simulink model "ADRC_Missile_Pitch"  (R2025b)
settings: Solver=VariableStepAuto  StartTime=0.0  StopTime=10.0  RelTol=1e-3
values from neighbouring files (symbols this model uses):
  b0 = adrc.b0    [adrc_controller.m]    (also in adrc_missile.m = 826.875; build_missile_pitch_model.m = 1; eso_observer.m)
  kp = wc^2    (= 64)    [adrc_missile.m]    (also in create_complete_missile_ADRC_simulink.m = wc^2; simulate_6DOF_ADRC.m)
settings Model: Creator=91872  LastModifiedBy=91872

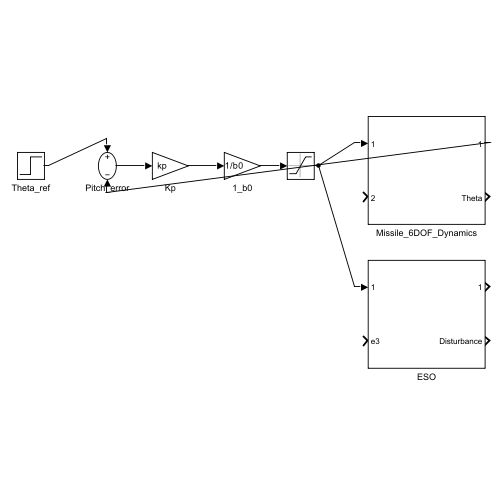
[thumbnail: Simulink's stored preview of the top-level diagram]
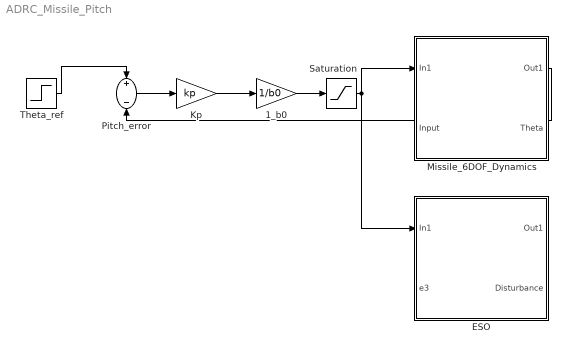
== system ADRC_Missile_Pitch ==
  1_b0 : Gain  Gain=1/b0
  ESO : Subsystem
  Kp : Gain  Gain=kp
  Missile_6DOF_Dynamics : Subsystem
  Pitch_error : Sum  Inputs=+-
  Saturation : Saturate  UpperLimit=0.4  LowerLimit=-0.4
  Theta_ref : Step  SampleTime=0
  wires:
  Theta_ref/1 -> Pitch_error/1
  Pitch_error/1 -> Kp/1
  Kp/1 -> 1_b0/1
  1_b0/1 -> Saturation/1
  Saturation/1 -> Missile_6DOF_Dynamics/1(In1), ESO/1(In1)
  Missile_6DOF_Dynamics/1(Out1) -> Pitch_error/2

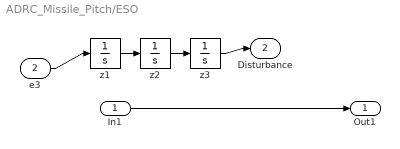
== system ADRC_Missile_Pitch/ESO ==
  In1 : Inport
  e3 : Inport  Port=2
  z1 : Integrator
  z2 : Integrator
  z3 : Integrator
  Out1 : Outport
  Disturbance : Outport  Port=2
  wires:
  In1/1 -> Out1/1
  e3/1 -> z1/1
  z1/1 -> z2/1
  z2/1 -> z3/1
  z3/1 -> Disturbance/1

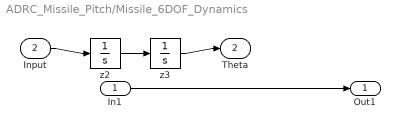
== system ADRC_Missile_Pitch/Missile_6DOF_Dynamics ==
  In1 : Inport
  Input : Inport  Port=2
  z2 : Integrator
  z3 : Integrator
  Out1 : Outport
  Theta : Outport  Port=2
  wires:
  In1/1 -> Out1/1
  Input/1 -> z2/1
  z2/1 -> z3/1
  z3/1 -> Theta/1
